simulink model "ControlPendulo2GDL_PNL_RE"  (R2019b)
settings: Solver=ode45  StartTime=0.0  StopTime=ts  RelTol=1e-3
values from neighbouring files (symbols this model uses):
  b1 = c8    (= 0.01)    [PenduloDatos.m]
  b2 = c8    (= 0.01)    [PenduloDatos.m]
  C = [1 0 0 0]    [PenduloDatos.m]
  g = 9.78    [PenduloDatos.m]
  I1 = 1/12*m1*(a1^2+d1^2)    (= 3.14166666667e-05)    [PenduloDatos.m]
  I2 = 1/12*m2*(a2^2+d2^2)    (= 1.20833333333e-05)    [PenduloDatos.m]
  K = place(Al,Bl,[Pd1 Pd2 Pd3 Pd4])    [PenduloDatos.m]
  K0 = inv(C*(inv(-Al+Bl*K))*Bl)    [PenduloDatos.m]
  l1 = c1    (= 0.3)    [PenduloDatos.m]
  l2 = c2    (= 0.2)    [PenduloDatos.m]
  lc1 = 0.25    [PenduloDatos.m]
  lc2 = 0.11    [PenduloDatos.m]
  m1 = c3    (= 0.065)    [PenduloDatos.m]
  m2 = c4    (= 0.025)    [PenduloDatos.m]
  U0 = [Tau1]    [PenduloDatos.m]
  X0 = [Tt1;Tpt1;Tt2;Tpt2]    [PenduloDatos.m]
libraries: simulink x1
settings Model: Creator=ARQ SEVILLA R  LastModifiedBy=ARQ SEVILLA R
settings SolverCC: AlgebraicLoopSolver=LineSearch

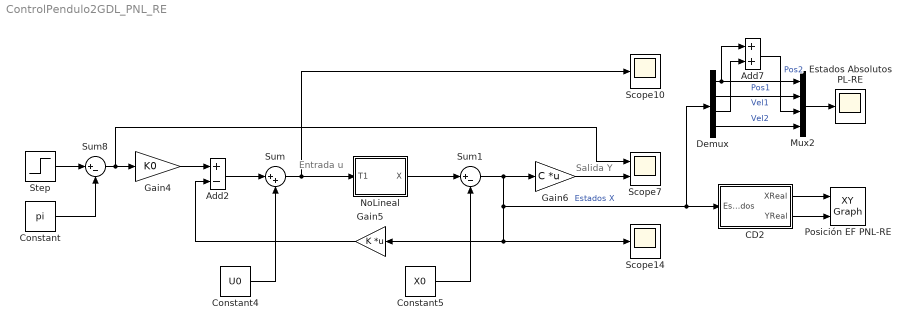
== system ControlPendulo2GDL_PNL_RE ==
  note: Entrada u
  note: Salida Y
  Add2 : Sum  Inputs=+-
  Add7 : Sum
  CD2 : Subsystem  TreatAsAtomicUnit=on
  Constant : Constant  Value=pi
  Constant4 : Constant  Value=U0
  Constant5 : Constant  Value=X0
  Demux : Demux
  Estados Absolutos PL-RE : Scope
  Gain4 : Gain  Gain=K0
  Gain5 : Gain  Gain=K  Multiplication=Matrix(K*u)
  Gain6 : Gain  Gain=C  Multiplication=Matrix(K*u)
  Mux2 : Mux
  NoLineal : Subsystem
  Posición EF PNL-RE : simulink/Sinks/XY Graph  xmin=-l2-l1  xmax=l2+l1  ymin=-l2-l1  ymax=l2+l1  st=-1
  Scope10 : Scope
  Scope14 : Scope
  Scope7 : Scope  NumInputPorts=2
  Step : Step  Time=0  After=pi+0.5  SampleTime=0
  Sum : Sum  Inputs=|++
  Sum1 : Sum  Inputs=|+-
  Sum8 : Sum  Inputs=|+-
  wires:
  Constant/1 -> Sum8/2
  Sum8/1 -> Gain4/1, Scope7/1
  Demux/1 -> Add7/1, Mux2/1  "Pos1"
  Gain5/1 -> Add2/2
  CD2/1(XReal) -> Posición EF PNL-RE/1
  Demux/3 -> Add7/2
  Add2/1 -> Sum/1
  Demux/4 -> Mux2/4  "Vel2"
  Sum1/1 -> Demux/1, CD2/1(Estados), Scope14/1, Gain5/1, Gain6/1  "Estados X"
  Gain6/1 -> Scope7/2
  Add7/1 -> Mux2/3  "Pos2"
  Step/1 -> Sum8/1
  Gain4/1 -> Add2/1
  Demux/2 -> Mux2/2  "Vel1"
  Constant4/1 -> Sum/2
  Mux2/1 -> Estados Absolutos PL-RE/1
  Sum/1 -> NoLineal/1(T1), Scope10/1
  Constant5/1 -> Sum1/2
  CD2/2(YReal) -> Posición EF PNL-RE/2
  NoLineal/1(X) -> Sum1/1

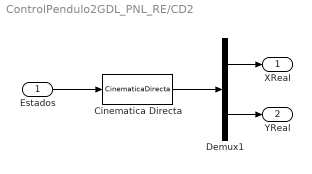
== system ControlPendulo2GDL_PNL_RE/CD2 ==
  Estados : Inport
  Cinematica Directa : MATLABFcn  MATLABFcn=CinematicaDirecta  OutputDimensions=2
  Demux1 : Demux  Outputs=2
  XReal : Outport  VectorParamsAs1DForOutWhenUnconnected=off
  YReal : Outport  Port=2  VectorParamsAs1DForOutWhenUnconnected=off
  wires:
  Cinematica Directa/1 -> Demux1/1
  Demux1/1 -> XReal/1
  Demux1/2 -> YReal/1
  Estados/1 -> Cinematica Directa/1

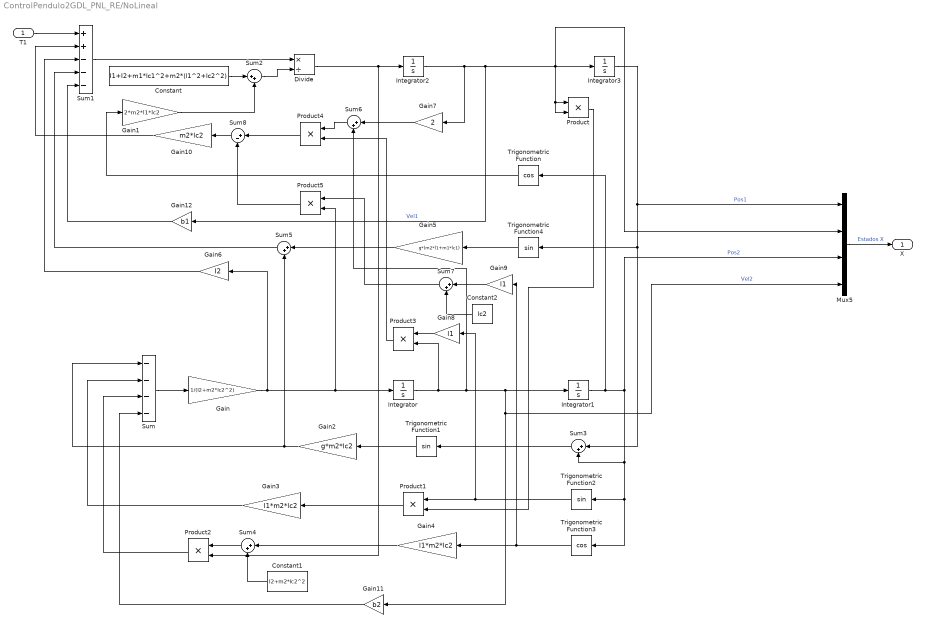
== system ControlPendulo2GDL_PNL_RE/NoLineal ==
  T1 : Inport
  Constant : Constant  Value=I1+I2+m1*lc1^2+m2*(l1^2+lc2^2)
  Constant1 : Constant  Value=I2+m2*lc2^2
  Constant2 : Constant  Value=lc2
  Divide : Product  Inputs=*/
  Gain : Gain  Gain=1/(I2+m2*lc2^2)
  Gain1 : Gain  Gain=2*m2*l1*lc2
  Gain10 : Gain  Gain=m2*lc2
  Gain11 : Gain  Gain=b2
  Gain12 : Gain  Gain=b1
  Gain2 : Gain  Gain=g*m2*lc2
  Gain3 : Gain  Gain=l1*m2*lc2
  Gain4 : Gain  Gain=l1*m2*lc2
  Gain5 : Gain  Gain=g*(m2*l1+m1*lc1)
  Gain6 : Gain  Gain=I2
  Gain7 : Gain  Gain=2
  Gain8 : Gain  Gain=l1
  Gain9 : Gain  Gain=l1
  Integrator : Integrator  InitialCondition=X0(4)
  Integrator1 : Integrator  InitialCondition=X0(3)
  Integrator2 : Integrator  InitialCondition=X0(2)
  Integrator3 : Integrator  InitialCondition=X0(1)
  Mux5 : Mux
  Product{,1..5} (6 alike) : Product
  Sum : Sum  Inputs=----
  Sum1 : Sum  Inputs=++---
  Sum{2..7} (6 alike) : Sum  Inputs=|++
  Sum8 : Sum  Inputs=|+-
  Trigonometric Function : Trigonometry  Operator=cos
  Trigonometric Function1 : Trigonometry
  Trigonometric Function2 : Trigonometry
  Trigonometric Function3 : Trigonometry  Operator=cos
  Trigonometric Function4 : Trigonometry
  X : Outport  VectorParamsAs1DForOutWhenUnconnected=off
  wires:
  Integrator/1 -> Product3/2, Gain11/1, Mux5/4, Integrator1/1, Sum6/2  "Vel2"
  Product4/1 -> Sum8/1
  Gain10/1 -> Sum1/2
  Constant/1 -> Sum2/1
  Sum7/1 -> Product5/1
  Sum1/1 -> Divide/1
  Gain6/1 -> Sum1/3
  Integrator1/1 -> Trigonometric Function/1, Mux5/3, Trigonometric Function3/1, Trigonometric Function2/1, Sum3/2  "Pos2"
  Sum3/1 -> Trigonometric Function1/1
  Gain11/1 -> Sum/4
  Product/1 -> Product1/2
  Gain4/1 -> Sum4/1
  Sum/1 -> Gain/1
  Constant2/1 -> Sum7/2
  Gain8/1 -> Product3/1
  Trigonometric Function3/1 -> Gain9/1, Gain4/1
  Product1/1 -> Gain3/1
  Gain7/1 -> Sum6/1
  Trigonometric Function2/1 -> Gain8/1, Product1/1
  Sum8/1 -> Gain10/1
  Gain2/1 -> Sum5/2, Sum/1
  Constant1/1 -> Sum4/2
  Integrator2/1 -> Gain7/1, Integrator3/1, Mux5/2, Product/2, Product/1, Gain12/1  "Vel1"
  Trigonometric Function4/1 -> Gain5/1
  Divide/1 -> Product2/2, Integrator2/1
  Product5/1 -> Sum8/2
  Gain3/1 -> Sum/2
  Gain9/1 -> Sum7/1
  T1/1 -> Sum1/1
  Gain/1 -> Product5/2, Integrator/1, Gain6/1
  Product3/1 -> Product4/2
  Sum2/1 -> Divide/2
  Sum6/1 -> Product4/1
  Integrator3/1 -> Mux5/1, Sum3/1, Trigonometric Function4/1  "Pos1"
  Trigonometric Function/1 -> Gain1/1
  Gain1/1 -> Sum2/2
  Sum5/1 -> Sum1/4
  Gain5/1 -> Sum5/1
  Gain12/1 -> Sum1/5
  Product2/1 -> Sum/3
  Sum4/1 -> Product2/1
  Trigonometric Function1/1 -> Gain2/1
  Mux5/1 -> X/1  "Estados X"
